simulink model "untitled"  (R2015a)
settings: Solver=ode45  StartTime=0.0  StopTime=20  RelTol=1e-3
values from neighbouring files (symbols this model uses):
  vmax = 200    [FullSys.m]    (also in FullSys4.m; Untitled.m)
  wn = sqrt(39.478)    [Untitled.m]
  xd = 1    [Untitled.m]
  xi = b/(2*wn)    [Untitled.m]
libraries: simulink x5
settings Model: Creator=Gabriel Garcia  LastModifiedBy=Gabriel Garcia

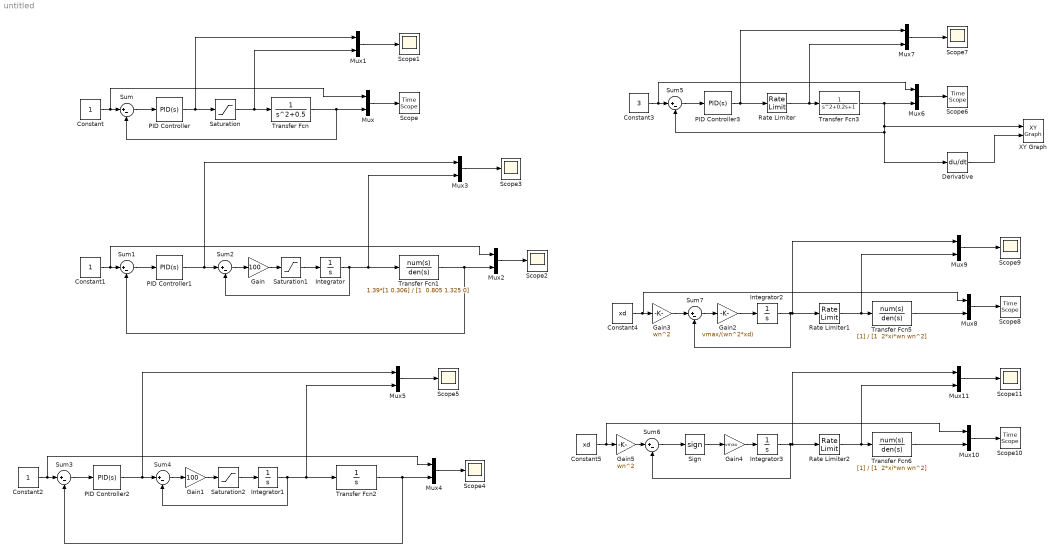
== system untitled ==
  Constant : Constant
  Constant1 : Constant
  Constant2 : Constant
  Constant3 : Constant  Value=3
  Constant4 : Constant  Value=xd
  Constant5 : Constant  Value=xd
  Derivative : Derivative
  Gain : Gain  Gain=100
  Gain1 : Gain  Gain=100
  Gain2 : Gain  Gain=vmax/(wn^2*xd)
  Gain3 : Gain  Gain=wn^2
  Gain4 : Gain  Gain=vmax
  Gain5 : Gain  Gain=wn^2
  Integrator{,1..3} (4 alike) : Integrator
  Mux{,1..11} (12 alike) : Mux  Inputs=2
  PID Controller : simulink/Continuous/PID Controller  Controller=PID  TimeDomain=Continuous-time  SampleTime=-1  IntegratorMethod=Forward Euler  FilterMethod=Forward Euler  Form=Parallel  UseFilter=on  ControllerParametersSource=internal  P=8  I=0  D=0  N=100  InitialConditionSource=internal  InitialConditionForIntegrator=0  InitialConditionForFilter=0  ExternalReset=none  LimitOutput=off  UpperSaturationLimit=inf  LowerSaturationLimit=-inf  LinearizeAsGain=on  AntiWindupMode=none  Kb=1  TrackingMode=off  Kt=1  PParamMin=[]  PParamMax=[]  IParamMin=[]  IParamMax=[]  DParamMin=[]  DParamMax=[]  NParamMin=[]  NParamMax=[]  KbParamMin=[]  KbParamMax=[]  KtParamMin=[]  KtParamMax=[]  POutMin=[]  POutMax=[]  IOutMin=[]  IOutMax=[]  DOutMin=[]  DOutMax=[]  NOutMin=[]  NOutMax=[]  KbOutMin=[]  KbOutMax=[]  KtOutMin=[]  KtOutMax=[]  IntegratorOutMin=[]  IntegratorOutMax=[]  FilterOutMin=[]  FilterOutMax=[]  SumOutMin=[]  SumOutMax=[]  SumI1OutMin=[]  SumI1OutMax=[]  SumI2OutMin=[]  SumI2OutMax=[]  SumI3OutMin=[]  SumI3OutMax=[]  SumDOutMin=[]  SumDOutMax=[]  SaturationOutMin=[]  SaturationOutMax=[]  IntegratorContinuousStateAttributes=''  IntegratorStateMustResolveToSignalObject=off  IntegratorRTWStateStorageClass=Auto  FilterContinuousStateAttributes=''  FilterStateMustResolveToSignalObject=off  FilterRTWStateStorageClass=Auto  DifferentiatorICPrevScaledInput=0  DifferentiatorOutMin=[]  DifferentiatorOutMax=[]
  PID Controller1 : simulink/Continuous/PID Controller  Controller=PID  TimeDomain=Continuous-time  SampleTime=-1  IntegratorMethod=Forward Euler  FilterMethod=Forward Euler  Form=Parallel  UseFilter=on  ControllerParametersSource=internal  P=10  I=0  D=0  N=100  InitialConditionSource=internal  InitialConditionForIntegrator=0  InitialConditionForFilter=0  ExternalReset=none  LimitOutput=off  UpperSaturationLimit=inf  LowerSaturationLimit=-inf  LinearizeAsGain=on  AntiWindupMode=none  Kb=1  TrackingMode=off  Kt=1  PParamMin=[]  PParamMax=[]  IParamMin=[]  IParamMax=[]  DParamMin=[]  DParamMax=[]  NParamMin=[]  NParamMax=[]  KbParamMin=[]  KbParamMax=[]  KtParamMin=[]  KtParamMax=[]  POutMin=[]  POutMax=[]  IOutMin=[]  IOutMax=[]  DOutMin=[]  DOutMax=[]  NOutMin=[]  NOutMax=[]  KbOutMin=[]  KbOutMax=[]  KtOutMin=[]  KtOutMax=[]  IntegratorOutMin=[]  IntegratorOutMax=[]  FilterOutMin=[]  FilterOutMax=[]  SumOutMin=[]  SumOutMax=[]  SumI1OutMin=[]  SumI1OutMax=[]  SumI2OutMin=[]  SumI2OutMax=[]  SumI3OutMin=[]  SumI3OutMax=[]  SumDOutMin=[]  SumDOutMax=[]  SaturationOutMin=[]  SaturationOutMax=[]  IntegratorContinuousStateAttributes=''  IntegratorStateMustResolveToSignalObject=off  IntegratorRTWStateStorageClass=Auto  FilterContinuousStateAttributes=''  FilterStateMustResolveToSignalObject=off  FilterRTWStateStorageClass=Auto  DifferentiatorICPrevScaledInput=0  DifferentiatorOutMin=[]  DifferentiatorOutMax=[]
  PID Controller2 : simulink/Continuous/PID Controller  Controller=PID  TimeDomain=Continuous-time  SampleTime=-1  IntegratorMethod=Forward Euler  FilterMethod=Forward Euler  Form=Parallel  UseFilter=on  ControllerParametersSource=internal  P=10  I=0  D=0  N=100  InitialConditionSource=internal  InitialConditionForIntegrator=0  InitialConditionForFilter=0  ExternalReset=none  LimitOutput=off  UpperSaturationLimit=inf  LowerSaturationLimit=-inf  LinearizeAsGain=on  AntiWindupMode=none  Kb=1  TrackingMode=off  Kt=1  PParamMin=[]  PParamMax=[]  IParamMin=[]  IParamMax=[]  DParamMin=[]  DParamMax=[]  NParamMin=[]  NParamMax=[]  KbParamMin=[]  KbParamMax=[]  KtParamMin=[]  KtParamMax=[]  POutMin=[]  POutMax=[]  IOutMin=[]  IOutMax=[]  DOutMin=[]  DOutMax=[]  NOutMin=[]  NOutMax=[]  KbOutMin=[]  KbOutMax=[]  KtOutMin=[]  KtOutMax=[]  IntegratorOutMin=[]  IntegratorOutMax=[]  FilterOutMin=[]  FilterOutMax=[]  SumOutMin=[]  SumOutMax=[]  SumI1OutMin=[]  SumI1OutMax=[]  SumI2OutMin=[]  SumI2OutMax=[]  SumI3OutMin=[]  SumI3OutMax=[]  SumDOutMin=[]  SumDOutMax=[]  SaturationOutMin=[]  SaturationOutMax=[]  IntegratorContinuousStateAttributes=''  IntegratorStateMustResolveToSignalObject=off  IntegratorRTWStateStorageClass=Auto  FilterContinuousStateAttributes=''  FilterStateMustResolveToSignalObject=off  FilterRTWStateStorageClass=Auto  DifferentiatorICPrevScaledInput=0  DifferentiatorOutMin=[]  DifferentiatorOutMax=[]
  PID Controller3 : simulink/Continuous/PID Controller  Controller=PID  TimeDomain=Continuous-time  SampleTime=-1  IntegratorMethod=Forward Euler  FilterMethod=Forward Euler  Form=Parallel  UseFilter=on  ControllerParametersSource=internal  P=1  I=0  D=0.04  N=100  InitialConditionSource=internal  InitialConditionForIntegrator=0  InitialConditionForFilter=0  ExternalReset=none  LimitOutput=off  UpperSaturationLimit=inf  LowerSaturationLimit=-inf  LinearizeAsGain=on  AntiWindupMode=none  Kb=1  TrackingMode=off  Kt=1  PParamMin=[]  PParamMax=[]  IParamMin=[]  IParamMax=[]  DParamMin=[]  DParamMax=[]  NParamMin=[]  NParamMax=[]  KbParamMin=[]  KbParamMax=[]  KtParamMin=[]  KtParamMax=[]  POutMin=[]  POutMax=[]  IOutMin=[]  IOutMax=[]  DOutMin=[]  DOutMax=[]  NOutMin=[]  NOutMax=[]  KbOutMin=[]  KbOutMax=[]  KtOutMin=[]  KtOutMax=[]  IntegratorOutMin=[]  IntegratorOutMax=[]  FilterOutMin=[]  FilterOutMax=[]  SumOutMin=[]  SumOutMax=[]  SumI1OutMin=[]  SumI1OutMax=[]  SumI2OutMin=[]  SumI2OutMax=[]  SumI3OutMin=[]  SumI3OutMax=[]  SumDOutMin=[]  SumDOutMax=[]  SaturationOutMin=[]  SaturationOutMax=[]  IntegratorContinuousStateAttributes=''  IntegratorStateMustResolveToSignalObject=off  IntegratorRTWStateStorageClass=Auto  FilterContinuousStateAttributes=''  FilterStateMustResolveToSignalObject=off  FilterRTWStateStorageClass=Auto  DifferentiatorICPrevScaledInput=0  DifferentiatorOutMin=[]  DifferentiatorOutMax=[]
  Rate Limiter : RateLimiter  RisingSlewLimit=7  FallingSlewLimit=-7  SampleTimeMode=inherited
  Rate Limiter1 : RateLimiter  RisingSlewLimit=vmax  FallingSlewLimit=-vmax  SampleTimeMode=inherited
  Rate Limiter2 : RateLimiter  RisingSlewLimit=vmax  FallingSlewLimit=-vmax  SampleTimeMode=inherited
  Saturation : Saturate  UpperLimit=5  LowerLimit=-5
  Saturation1 : Saturate  UpperLimit=25  LowerLimit=-25
  Saturation2 : Saturate  UpperLimit=0.4  LowerLimit=-0.4
  Scope{,6,8,10} (4 alike) : TimeScope
  Scope{1..5,7,9,11} (8 alike) : Scope
      Scope11 settings: TimeRange=20  YMin=-1  YMax=9  SaveName=ScopeData11
      Scope2 settings: SaveName=ScopeData2
      Scope3 settings: SaveName=ScopeData3
      Scope4 settings: SaveName=ScopeData4
      Scope5 settings: SaveName=ScopeData5
      Scope7 settings: TimeRange=20  YMin=-1  YMax=9  SaveName=ScopeData7
      Scope9 settings: TimeRange=20  YMin=-1  YMax=9  SaveName=ScopeData9
  Sign : Signum  ZeroCross=off
  Sum{,1..7} (8 alike) : Sum  Inputs=|+-
  Transfer Fcn : TransferFcn  Denominator="[1  0 0.5]"
  Transfer Fcn1 : TransferFcn  Numerator=1.39*[1 0.306]  Denominator="[1  0.805 1.325 0]"
  Transfer Fcn2 : TransferFcn  Denominator=[1 0]
  Transfer Fcn3 : TransferFcn  Denominator="[1  0.2 1]"
  Transfer Fcn5 : TransferFcn  Denominator="[1  2*xi*wn wn^2]"
  Transfer Fcn6 : TransferFcn  Denominator="[1  2*xi*wn wn^2]"
  XY Graph : simulink/Sinks/XY Graph  xmin=-10  xmax=10  ymin=-10  ymax=10  st=-1
  wires:
  Mux/1 -> Scope/1
  PID Controller/1 -> Mux1/1, Saturation/1
  Saturation/1 -> Mux1/2, Transfer Fcn/1
  Constant/1 -> Mux/1, Sum/1
  Sum/1 -> PID Controller/1
  Transfer Fcn/1 -> Mux/2, Sum/2
  Mux1/1 -> Scope1/1
  Mux2/1 -> Scope2/1
  Constant1/1 -> Mux2/1, Sum1/1
  Sum1/1 -> PID Controller1/1
  Transfer Fcn1/1 -> Mux2/2, Sum1/2
  Mux3/1 -> Scope3/1
  Gain/1 -> Saturation1/1
  Saturation1/1 -> Integrator/1
  Sum2/1 -> Gain/1
  Integrator/1 -> Mux3/2, Transfer Fcn1/1, Sum2/2
  PID Controller1/1 -> Mux3/1, Sum2/1
  Mux4/1 -> Scope4/1
  Constant2/1 -> Mux4/1, Sum3/1
  Sum3/1 -> PID Controller2/1
  Transfer Fcn2/1 -> Mux4/2, Sum3/2
  Mux5/1 -> Scope5/1
  Gain1/1 -> Saturation2/1
  Saturation2/1 -> Integrator1/1
  Sum4/1 -> Gain1/1
  Integrator1/1 -> Mux5/2, Transfer Fcn2/1, Sum4/2
  PID Controller2/1 -> Mux5/1, Sum4/1
  Mux6/1 -> Scope6/1
  Constant3/1 -> Mux6/1, Sum5/1
  Sum5/1 -> PID Controller3/1
  Transfer Fcn3/1 -> Mux6/2, XY Graph/1, Derivative/1, Sum5/2
  Mux7/1 -> Scope7/1
  PID Controller3/1 -> Rate Limiter/1, Mux7/1
  Rate Limiter/1 -> Mux7/2, Transfer Fcn3/1
  Mux8/1 -> Scope8/1
  Constant4/1 -> Gain3/1, Mux8/1
  Transfer Fcn5/1 -> Mux8/2
  Mux9/1 -> Scope9/1
  Integrator2/1 -> Rate Limiter1/1, Mux9/1, Sum7/2
  Rate Limiter1/1 -> Mux9/2, Transfer Fcn5/1
  Sum7/1 -> Gain2/1
  Gain2/1 -> Integrator2/1
  Gain3/1 -> Sum7/1
  Mux10/1 -> Scope10/1
  Constant5/1 -> Gain5/1, Mux10/1
  Transfer Fcn6/1 -> Mux10/2
  Mux11/1 -> Scope11/1
  Integrator3/1 -> Rate Limiter2/1, Mux11/1, Sum6/2
  Rate Limiter2/1 -> Mux11/2, Transfer Fcn6/1
  Gain5/1 -> Sum6/1
  Sum6/1 -> Sign/1
  Gain4/1 -> Integrator3/1
  Sign/1 -> Gain4/1
  Derivative/1 -> XY Graph/2
